simulink model "SystemARMAX"  (R2015a)
settings: Solver=FixedStepDiscrete  StartTime=0.0  StopTime=Tend  FixedStep=Tp  RelTol=1e-3
values from neighbouring files (symbols this model uses):
  c1o = 0.99    [ZADANIE_1_2.m]    (also in ZADANIE_2_1.m = 0; Zad_1_1.m = 0; Zad_1_1_8_kolorowe.m; Zad_2_1_zapominanie.m = 0)
  Td = 1500    [ZADANIE_1_2.m]    (also in ZADANIE_2_1.m = 500; Zad_1_1.m; Zad_1_1_8_kolorowe.m; Zad_2_1_zapominanie.m = 500)
  Tp = 0.1    [ZADANIE_1_2.m]    (also in ZADANIE_2_1.m; Zad_1_1.m; Zad_1_1_8_kolorowe.m; Zad_2_1_zapominanie.m)
libraries: simulink x2
settings Model: CovExternalEMLEnable=on  Creator=mgmil  LastModifiedBy=mgmil
settings DataIOCC: SignalLoggingSaveFormat=ModelDataLogs
settings OptimizationCC: InitFltsAndDblsToZero=on
settings DebuggingCC: SaveWithParameterizedLinksMsg=none  UnderspecifiedInitializationDetection=Classic  MergeDetectMultiDrivingBlocksExec=none  SignalResolutionControl=TryResolveAllWithWarning  SolverPrmCheckMsg=warning  MultiTaskDSMMsg=warning  MultiTaskCondExecSysMsg=none  FcnCallInpInsideContextMsg=EnableAllAsWarning
settings SFSimCC: SimUseLocalCustomCode=on
settings RTWCC: RTWUseLocalCustomCode=on
settings GRTTargetCC: TargetFcnLib=ansi_tfl_tmw.mat  GeneratePreprocessorConditionals=Use local settings  CombineOutputUpdateFcns=off  GRTInterface=on

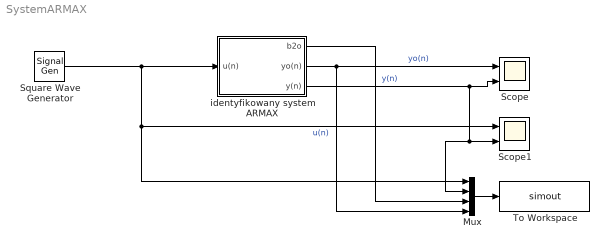
== system SystemARMAX ==
  Mux : Mux
  Scope : Scope  NumInputPorts=2
      settings: TimeRange=auto  MaxDataPoints=5000  SaveToWorkspace=off  YMin=-5.51861~-5  YMax=5.6277~5  SampleTime=-1
  Scope1 : Scope  NumInputPorts=2
      settings: TimeRange=auto  MaxDataPoints=5000  SaveToWorkspace=off  SaveName=ScopeData2  YMin=-5.51861~-5  YMax=5.6277~5  SampleTime=-1
  Square Wave Generator : SignalGenerator  WaveForm=square  Frequency=0.025
  To Workspace : ToWorkspace  VariableName=simout  SampleTime=-1
  identyfikowany system ARMAX : Subsystem
  wires:
  Square Wave Generator/1 -> Scope1/1, Mux/1, identyfikowany system ARMAX/1(u(n))  "u(n)"
  identyfikowany system ARMAX/2(yo(n)) -> Mux/4, Scope/1  "yo(n)"
  identyfikowany system ARMAX/3(y(n)) -> Mux/2, Scope1/2, Scope/2  "y(n)"
  Mux/1 -> To Workspace/1
  identyfikowany system ARMAX/1(b2o) -> Mux/3

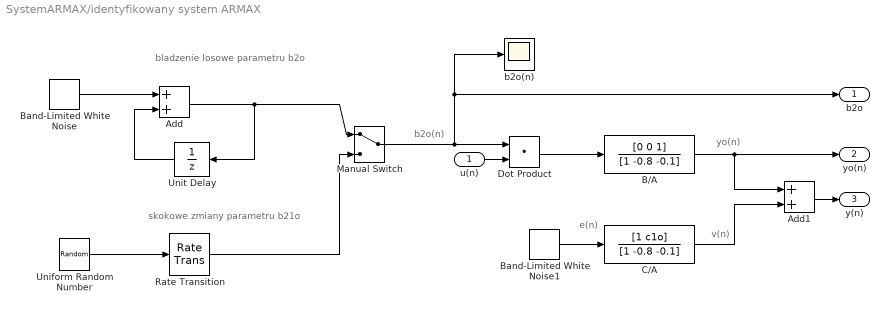
== system SystemARMAX/identyfikowany system ARMAX ==
  note: e(n)
  note: v(n)
  note: yo(n)
  note: b2o(n)
  note: skokowe zmiany parametru b21o
  note: bladzenie losowe parametru b2o
  u(n) : Inport
  Add : Sum
  Add1 : Sum
  B/A : DiscreteFilter  Numerator=[0 0 1]  Denominator=[1 -0.8 -0.1]  SampleTime=Tp
  Band-Limited White Noise : simulink/Sources/Band-Limited White Noise  Cov=[0.00001*Tp]  Ts=Tp  seed=[23341]
  Band-Limited White Noise1 : simulink/Sources/Band-Limited White Noise  Cov=[0.001*Tp]  Ts=Tp  seed=[23341]
  C/A : DiscreteFilter  Numerator=[1 c1o]  Denominator=[1 -0.8 -0.1]  SampleTime=Tp
  Dot Product : DotProduct  InputSameDT=on  OutDataTypeStr=Inherit: Inherit via internal rule
  Manual Switch : ManualSwitch
  Rate Transition : RateTransition  X0=0.5  OutPortSampleTime=Tp
  Uniform Random Number : UniformRandomNumber  Minimum=0.1  Maximum=0.8  Seed=2  SampleTime=Td
  Unit Delay : UnitDelay  SampleTime=Tp
  b2o(n) : Scope
      settings: TimeRange=auto  LimitDataPoints=on  MaxDataPoints=5000  SaveToWorkspace=off  SaveName=ScopeData  YMin=0.04339  YMax=0.50216  SampleTime=-1
  b2o : Outport
  yo(n) : Outport  Port=2
  y(n) : Outport  Port=3
  wires:
  Band-Limited White Noise/1 -> Add/1
  Add/1 -> Unit Delay/1, Manual Switch/1
  Unit Delay/1 -> Add/2
  Uniform Random Number/1 -> Rate Transition/1
  Rate Transition/1 -> Manual Switch/2
  Manual Switch/1 -> Dot Product/1, b2o/1, b2o(n)/1
  Dot Product/1 -> B/A/1
  C/A/1 -> Add1/2
  B/A/1 -> Add1/1, yo(n)/1
  Band-Limited White Noise1/1 -> C/A/1
  u(n)/1 -> Dot Product/2
  Add1/1 -> y(n)/1
